simulink model "CombinedModel"  (R2020a)
settings: Solver=FixedStepAuto  StartTime=0  StopTime=100  FixedStep=0.01  RelTol=1e-3
values from neighbouring files (symbols this model uses):
  delay = delay_Range(k)    [GainDelay3ParamSweep.m]    (also in GainFreq2ParamSweep.m = sim_Set.delay; GainFreq3ParamSweep.m = sim_Set.delay; stabChecker2GainDelay.m)
  PSA = gain_Range2(j)    [GainDelay3ParamSweep.m]    (also in GainFreq2ParamSweep.m = gain_Range(i); GainFreq3ParamSweep.m)
  PSA_sat_low = sim_Set.PSA_sat_low    [GainDelay3ParamSweep.m]    (also in GainFreq2ParamSweep.m; GainFreq3ParamSweep.m)
  PSA_sat_up = sim_Set.PSA_sat_up    [GainDelay3ParamSweep.m]    (also in GainFreq2ParamSweep.m; GainFreq3ParamSweep.m)
  PSM = gain_Range2(j)    [GainDelay3ParamSweep.m]    (also in GainFreq2ParamSweep.m = gain_Range(i); GainFreq3ParamSweep.m)
  PSM_sat_low = sim_Set.PSM_sat_low    [GainDelay3ParamSweep.m]    (also in GainFreq2ParamSweep.m; GainFreq3ParamSweep.m)
  PSM_sat_up = sim_Set.PSM_sat_up    [GainDelay3ParamSweep.m]    (also in GainFreq2ParamSweep.m; GainFreq3ParamSweep.m)
  vout_low = sim_Set.vout_low    [GainDelay3ParamSweep.m]    (also in GainFreq2ParamSweep.m; GainFreq3ParamSweep.m)
  vout_up = sim_Set.vout_up    [GainDelay3ParamSweep.m]    (also in GainFreq2ParamSweep.m; GainFreq3ParamSweep.m)
  VSA = gain_Range2(j)    [GainDelay3ParamSweep.m]    (also in GainFreq2ParamSweep.m = gain_Range(i); GainFreq3ParamSweep.m)
  VSA_sat_low = sim_Set.VSA_sat_low    [GainDelay3ParamSweep.m]    (also in GainFreq2ParamSweep.m; GainFreq3ParamSweep.m)
  VSA_sat_up = sim_Set.VSA_sat_up    [GainDelay3ParamSweep.m]    (also in GainFreq2ParamSweep.m; GainFreq3ParamSweep.m)
  VSM = gain_Range2(j)    [GainDelay3ParamSweep.m]    (also in GainFreq2ParamSweep.m = gain_Range(i); GainFreq3ParamSweep.m)
  VSM_sat_low = sim_Set.VSM_sat_low    [GainDelay3ParamSweep.m]    (also in GainFreq2ParamSweep.m; GainFreq3ParamSweep.m)
  VSM_sat_up = sim_Set.VSM_sat_up    [GainDelay3ParamSweep.m]    (also in GainFreq2ParamSweep.m; GainFreq3ParamSweep.m)
settings Model: Creator=Brock  LastModifiedBy=Brock

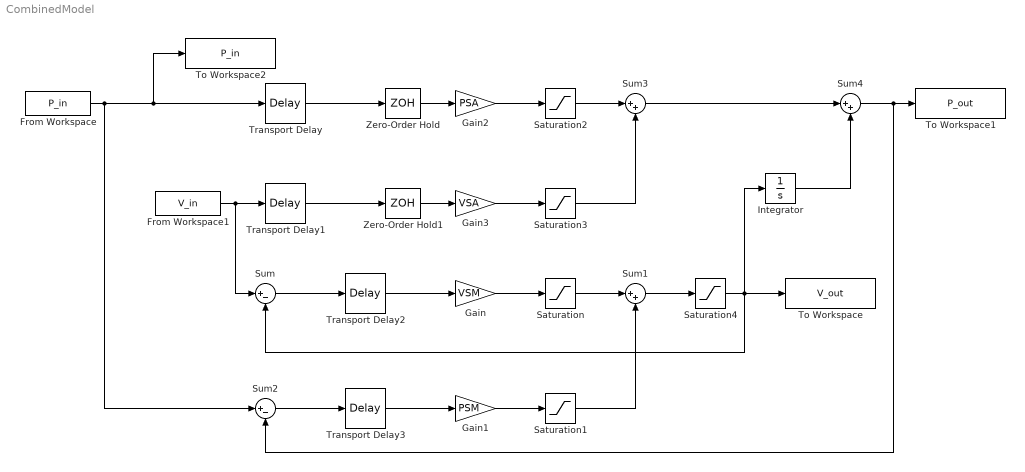
== system CombinedModel ==
  From Workspace : FromWorkspace  VariableName=P_in
  From Workspace1 : FromWorkspace  VariableName=V_in
  Gain : Gain  Gain=VSM
  Gain1 : Gain  Gain=PSM
  Gain2 : Gain  Gain=PSA
  Gain3 : Gain  Gain=VSA
  Integrator : Integrator
  Saturation : Saturate  UpperLimit=VSM_sat_up  LowerLimit=VSM_sat_low
  Saturation1 : Saturate  UpperLimit=PSM_sat_up  LowerLimit=PSM_sat_low
  Saturation2 : Saturate  UpperLimit=PSA_sat_up  LowerLimit=PSA_sat_low
  Saturation3 : Saturate  UpperLimit=VSA_sat_up  LowerLimit=VSA_sat_low
  Saturation4 : Saturate  UpperLimit=vout_up  LowerLimit=vout_low
  Sum : Sum  Inputs=|+-
  Sum1 : Sum  Inputs=|++
  Sum2 : Sum  Inputs=|+-
  Sum3 : Sum  Inputs=|++
  Sum4 : Sum  Inputs=|++
  To Workspace : ToWorkspace  VariableName=V_out  SampleTime=-1
  To Workspace1 : ToWorkspace  VariableName=P_out  SampleTime=-1
  To Workspace2 : ToWorkspace  VariableName=P_in  SampleTime=-1
  Transport Delay{,1..3} (4 alike) : TransportDelay  DelayTime=delay
  Zero-Order Hold : ZeroOrderHold  SampleTime=delay
  Zero-Order Hold1 : ZeroOrderHold  SampleTime=delay
  wires:
  From Workspace/1 -> Sum2/1, To Workspace2/1, Transport Delay/1
  From Workspace1/1 -> Sum/1, Transport Delay1/1
  Sum/1 -> Transport Delay2/1
  Transport Delay/1 -> Zero-Order Hold/1
  Transport Delay1/1 -> Zero-Order Hold1/1
  Transport Delay2/1 -> Gain/1
  Gain/1 -> Saturation/1
  Saturation/1 -> Sum1/1
  Sum2/1 -> Transport Delay3/1
  Transport Delay3/1 -> Gain1/1
  Gain1/1 -> Saturation1/1
  Saturation1/1 -> Sum1/2
  Zero-Order Hold/1 -> Gain2/1
  Zero-Order Hold1/1 -> Gain3/1
  Gain3/1 -> Saturation3/1
  Gain2/1 -> Saturation2/1
  Saturation2/1 -> Sum3/1
  Saturation3/1 -> Sum3/2
  Sum3/1 -> Sum4/1
  Integrator/1 -> Sum4/2
  Sum4/1 -> Sum2/2, To Workspace1/1
  Sum1/1 -> Saturation4/1
  Saturation4/1 -> To Workspace/1, Sum/2, Integrator/1
